simulink model "Standard_Treatment_Include_IVdextrose_IVinsulin_carbs"  (Simulink 7.5)
settings: Solver=ode45  StartTime=0.0  StopTime=10.0  RelTol=1e-3
undefined symbols (not defined in the file or in its folder): ctrller
settings Model: Creator=sriddle  LastModifiedBy=sriddle

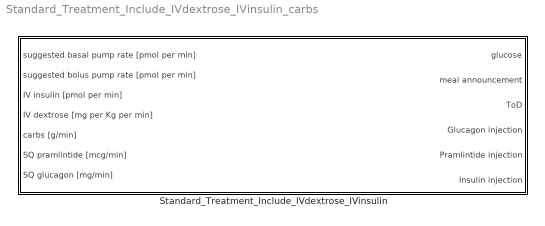
== system Standard_Treatment_Include_IVdextrose_IVinsulin_carbs ==
  Standard_Treatment_Include_IVdextrose_IVinsulin : Subsystem

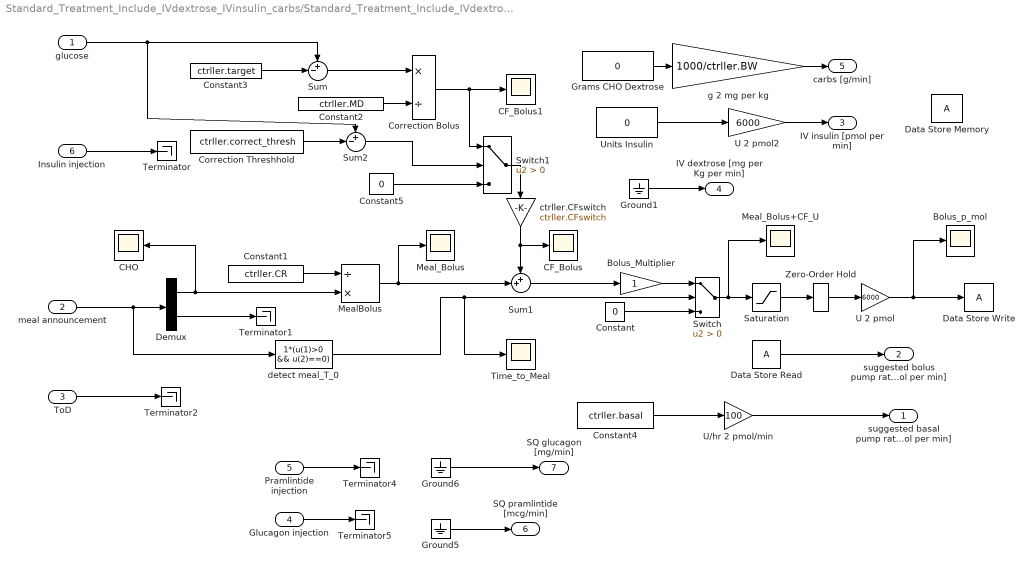
== system Standard_Treatment_Include_IVdextrose_IVinsulin_carbs/Standard_Treatment_Include_IVdextrose_IVinsulin ==
  glucose : Inport  OutDataType=sfix(16)  OutScaling=2^0
  meal announcement : Inport  Port=2  OutDataType=sfix(16)  OutScaling=2^0
  ToD : Inport  Port=3  OutDataType=sfix(16)  OutScaling=2^0
  Glucagon injection : Inport  Port=4
  Pramlintide injection : Inport  Port=5
  Insulin injection : Inport  Port=6  OutDataType=sfix(16)  OutScaling=2^0
  Bolus_Multiplier : Gain  ParameterDataType=fixdt(1, 16)  ParameterScaling=2^0  OutDataType=fixdt(1, 16)  OutScaling=2^0
  Bolus_p_mol : Scope
      settings: YMin=0  YMax=60000  SaveName=ScopeData5
  CF_Bolus : Scope
      settings: SaveName=ScopeData15
  CF_Bolus1 : Scope
      settings: SaveName=ScopeData18
  CHO : Scope
      settings: YMin=0  YMax=0.01
  Constant : Constant  Value=0  OutDataType=sfix(16)  OutScaling=2^0
  Constant1 : Constant  Value=ctrller.CR  OutDataType=sfix(16)  OutScaling=2^0
  Constant2 : Constant  Value=ctrller.MD  OutDataType=sfix(16)  OutScaling=2^0
  Constant3 : Constant  Value=ctrller.target  OutDataType=sfix(16)  OutScaling=2^0
  Constant4 : Constant  Value=ctrller.basal  OutDataType=sfix(16)  OutScaling=2^0
  Constant5 : Constant  Value=0  OutDataType=sfix(16)  OutScaling=2^0
  Correction Bolus : Product  Inputs=*/  OutDataType=sfix(16)  OutScaling=2^-10
  Correction Threshhold : Constant  Value=ctrller.correct_thresh  OutDataType=sfix(16)  OutScaling=2^0
  Data Store Memory : DataStoreMemory  DataStoreName=A  ReadBeforeWriteMsg=warning  WriteAfterWriteMsg=warning  WriteAfterReadMsg=warning  OutDataType=fixdt(1, 16)  OutScaling=2^0
  Data Store Read : DataStoreRead  DataStoreName=A  SampleTime=0
  Data Store Write : DataStoreWrite  DataStoreName=A  SampleTime=-1
  Demux : Demux  Outputs=2
  Grams CHO Dextrose : Constant  Value=0  OutDataType=fixdt(1, 16)  OutScaling=2^0
  Ground1 : Ground
  Ground5 : Ground
  Ground6 : Ground
  MealBolus : Product  Inputs=/*  OutDataType=sfix(16)  OutScaling=2^-10
  Meal_Bolus : Scope
      settings: SaveName=ScopeData10
  Meal_Bolus+CF_U : Scope
      settings: YMin=0  YMax=3000  SaveName=ScopeData2
  Saturation : Saturate  UpperLimit=100  LowerLimit=0  OutDataType=fixdt(1, 16)  OutScaling=2^0
  Sum : Sum  Inputs=+-|  OutDataType=sfix(16)  OutScaling=2^0
  Sum1 : Sum  Inputs=++|  OutDataType=sfix(16)  OutScaling=2^0
  Sum2 : Sum  Inputs=+-|  OutDataType=sfix(16)  OutScaling=2^0
  Switch : Switch  Criteria=u2 > Threshold  OutDataType=sfix(16)  OutScaling=2^0
  Switch1 : Switch  Criteria=u2 > Threshold  OutDataType=sfix(16)  OutScaling=2^0
  Terminator{,1..2,4..5} (5 alike) : Terminator
  Time_to_Meal : Scope
      settings: SaveName=ScopeData3
  U 2 pmol : Gain  Gain=6000  ParameterDataType=sfix(16)  ParameterScaling=2^0  OutDataType=sfix(16)  OutScaling=2^0
  U 2 pmol2 : Gain  Gain=6000  ParameterDataType=fixdt(1, 16)  ParameterScaling=2^0  OutDataType=fixdt(1, 16)  OutScaling=2^0
  U/hr 2 pmol/min : Gain  Gain=100  ParameterDataType=sfix(16)  ParameterScaling=2^0  OutDataType=sfix(16)  OutScaling=2^0
  Units Insulin : Constant  Value=0  OutDataType=fixdt(1, 16)  OutScaling=2^0
  Zero-Order Hold : ZeroOrderHold
  ctrller.CFswitch : Gain  Gain=ctrller.CFswitch  ParameterDataType=fixdt(1, 16)  ParameterScaling=2^0  OutDataType=fixdt(1, 16)  OutScaling=2^0
  detect meal_T_0 : Fcn  Expr=1*(u(1)>0 && u(2)==0)
  g 2 mg per kg : Gain  Gain=1000/ctrller.BW  ParameterDataType=fixdt(1, 16)  ParameterScaling=2^0  OutDataType=fixdt(1, 16)  OutScaling=2^0
  suggested basal pump rate [pmol per min] : Outport  OutDataType=sfix(16)  OutScaling=2^0
  suggested bolus pump rate [pmol per min] : Outport  Port=2  OutDataType=sfix(16)  OutScaling=2^0
  IV insulin [pmol per min] : Outport  Port=3  OutDataType=sfix(16)  OutScaling=2^0
  IV dextrose [mg per Kg per min] : Outport  Port=4  OutDataType=sfix(16)  OutScaling=2^0
  carbs [g/min] : Outport  Port=5  OutDataType=sfix(16)  OutScaling=2^0
  SQ pramlintide [mcg/min] : Outport  Port=6
  SQ glucagon [mg/min] : Outport  Port=7
  wires:
  Ground1/1 -> IV dextrose [mg per Kg per min]/1
  Data Store Read/1 -> suggested bolus pump rate [pmol per min]/1
  U 2 pmol/1 -> Data Store Write/1, Bolus_p_mol/1
  Zero-Order Hold/1 -> U 2 pmol/1
  Sum2/1 -> Switch1/2
  Correction Threshhold/1 -> Sum2/2
  Constant5/1 -> Switch1/3
  Switch1/1 -> ctrller.CFswitch/1
  Correction Bolus/1 -> CF_Bolus1/1, Switch1/1
  Constant4/1 -> U/hr 2 pmol/min/1
  Sum1/1 -> Bolus_Multiplier/1
  MealBolus/1 -> Sum1/2, Meal_Bolus/1
  Constant2/1 -> Correction Bolus/2
  Sum/1 -> Correction Bolus/1
  Constant3/1 -> Sum/2
  Constant/1 -> Switch/3
  detect meal_T_0/1 -> Switch/2, Time_to_Meal/1
  ToD/1 -> Terminator2/1
  Insulin injection/1 -> Terminator/1
  glucose/1 -> Sum/1, Sum2/1
  Constant1/1 -> MealBolus/1
  ctrller.CFswitch/1 -> Sum1/1, CF_Bolus/1
  Demux/1 -> MealBolus/2, CHO/1
  meal announcement/1 -> Demux/1, detect meal_T_0/1
  Saturation/1 -> Zero-Order Hold/1
  Switch/1 -> Saturation/1, Meal_Bolus+CF_U/1
  Demux/2 -> Terminator1/1
  Grams CHO Dextrose/1 -> g 2 mg per kg/1
  U 2 pmol2/1 -> IV insulin [pmol per min]/1
  Units Insulin/1 -> U 2 pmol2/1
  U/hr 2 pmol/min/1 -> suggested basal pump rate [pmol per min]/1
  g 2 mg per kg/1 -> carbs [g/min]/1
  Bolus_Multiplier/1 -> Switch/1
  Pramlintide injection/1 -> Terminator4/1
  Glucagon injection/1 -> Terminator5/1
  Ground6/1 -> SQ glucagon [mg/min]/1
  Ground5/1 -> SQ pramlintide [mcg/min]/1
